simulink model "Cardiovs_Perez22210425"  (R2023a)
settings: Solver=ode15s  StartTime=0.0  StopTime=10  MaxStep=1e-3  RelTol=1e-3
settings Model: Creator=najap  LastModifiedBy=najap
settings DataIOCC: SaveOutput=off  ReturnWorkspaceOutputs=off  TimeSaveName=t
settings DebuggingCC: AlgebraicLoopMsg=none  ArtificialAlgebraicLoopMsg=none  MaxConsecutiveZCsMsg=none  SolverPrmCheckMsg=warning  ModelReferenceExtraNoncontSigs=none  OperatingPointInterfaceChecksumMismatchMsg=none

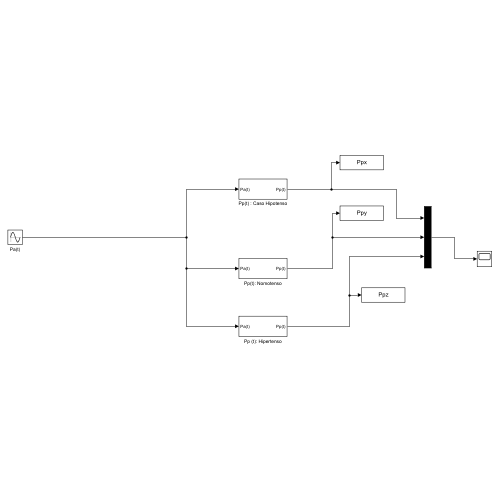
[thumbnail: Simulink's stored preview of the top-level diagram]
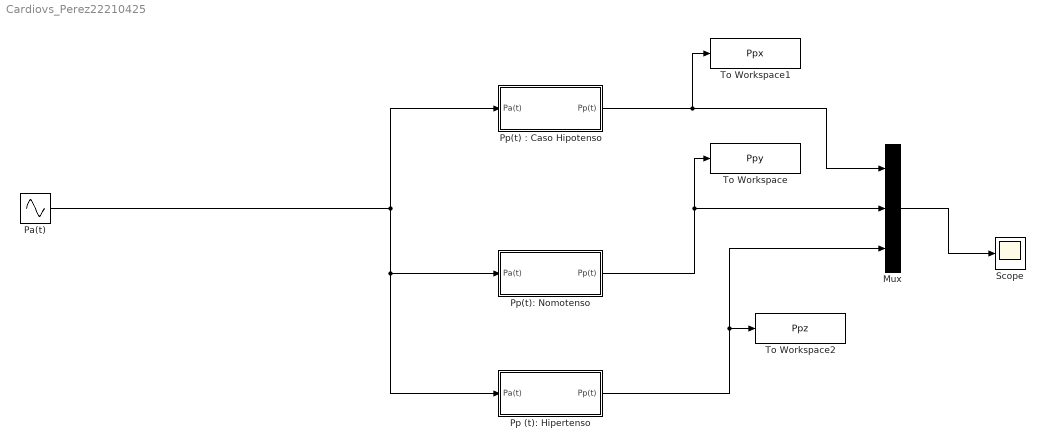
== system Cardiovs_Perez22210425 ==
  Mux : Mux  Inputs=3
  Pa(t) : Sin  Bias=0.8  Frequency=2*pi*95/60  SampleTime=0
  Pp (t): Hipertenso : Subsystem
  "Pp(t) : Caso Hipotenso" : Subsystem
  Pp(t): Nomotenso : Subsystem
  Scope : Scope
  To Workspace : ToWorkspace  VariableName=Ppy  SaveFormat=Timeseries  SampleTime=-1
  To Workspace1 : ToWorkspace  VariableName=Ppx  SaveFormat=Timeseries  SampleTime=-1
  To Workspace2 : ToWorkspace  VariableName=Ppz  SaveFormat=Timeseries  SampleTime=-1
  wires:
  Mux/1 -> Scope/1
  Pp (t): Hipertenso/1(Pp(t)) -> Mux/3, To Workspace2/1
  Pa(t)/1 -> Pp(t): Nomotenso/1(Pa(t)), Pp (t): Hipertenso/1(Pa(t)), "Pp(t) : Caso Hipotenso"/1(Pa(t))
  Pp(t): Nomotenso/1(Pp(t)) -> To Workspace/1, Mux/2
  "Pp(t) : Caso Hipotenso"/1(Pp(t)) -> To Workspace1/1, Mux/1

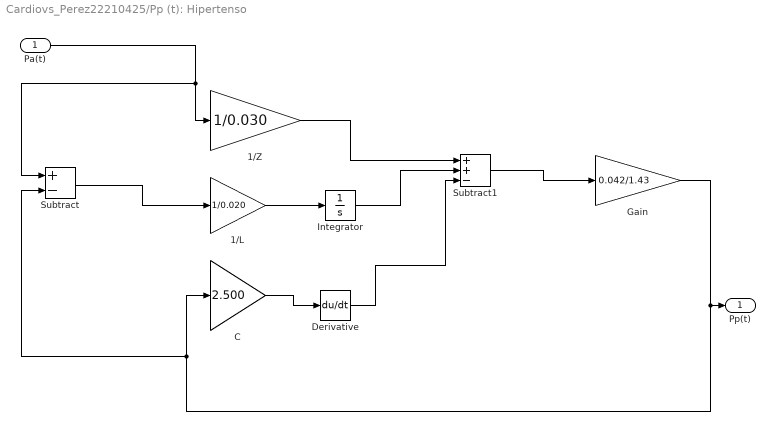
== system Cardiovs_Perez22210425/Pp (t): Hipertenso ==
  Pa(t) : Inport
  1/L : Gain  Gain=1/0.020
  1/Z : Gain  Gain=1/0.030
  C : Gain  Gain=2.500
  Derivative : Derivative
  Gain : Gain  Gain=0.042/1.43
  Integrator : Integrator
  Subtract : Sum  Inputs=+-
  Subtract1 : Sum  Inputs=++-
  Pp(t) : Outport
  wires:
  Gain/1 -> Pp(t)/1, Subtract/2, C/1
  1/Z/1 -> Subtract1/1
  Subtract1/1 -> Gain/1
  Integrator/1 -> Subtract1/2
  Subtract/1 -> 1/L/1
  1/L/1 -> Integrator/1
  Derivative/1 -> Subtract1/3
  C/1 -> Derivative/1
  Pa(t)/1 -> Subtract/1, 1/Z/1

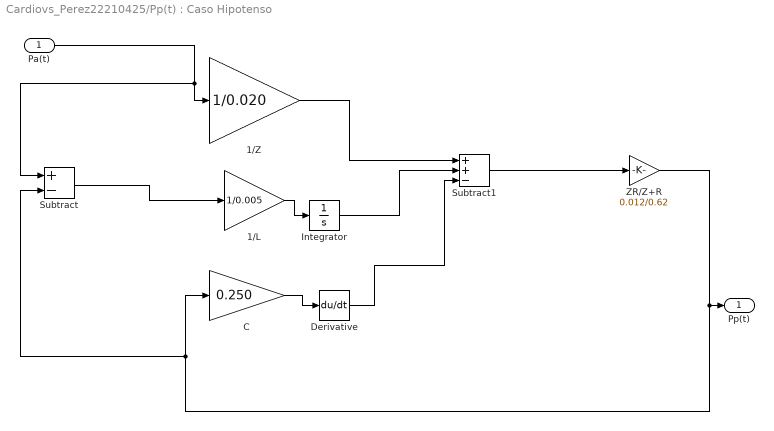
== system Cardiovs_Perez22210425/Pp(t) : Caso Hipotenso ==
  Pa(t) : Inport
  1/L : Gain  Gain=1/0.005
  1/Z : Gain  Gain=1/0.020
  C : Gain  Gain=0.250
  Derivative : Derivative
  Integrator : Integrator
  Subtract : Sum  Inputs=+-
  Subtract1 : Sum  Inputs=++-
  ZR/Z+R : Gain  Gain=0.012/0.62
  Pp(t) : Outport
  wires:
  C/1 -> Derivative/1
  1/L/1 -> Integrator/1
  Integrator/1 -> Subtract1/2
  1/Z/1 -> Subtract1/1
  Derivative/1 -> Subtract1/3
  Subtract/1 -> 1/L/1
  Pa(t)/1 -> Subtract/1, 1/Z/1
  Subtract1/1 -> ZR/Z+R/1
  ZR/Z+R/1 -> Subtract/2, C/1, Pp(t)/1

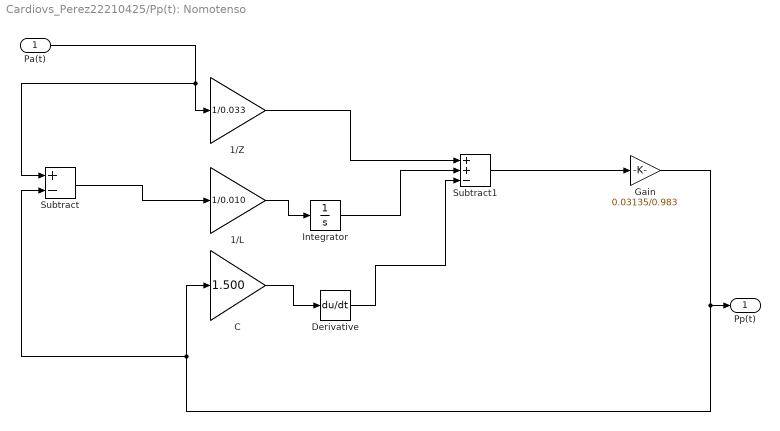
== system Cardiovs_Perez22210425/Pp(t): Nomotenso ==
  Pa(t) : Inport
  1/L : Gain  Gain=1/0.010
  1/Z : Gain  Gain=1/0.033
  C : Gain  Gain=1.500
  Derivative : Derivative
  Gain : Gain  Gain=0.03135/0.983
  Integrator : Integrator
  Subtract : Sum  Inputs=+-
  Subtract1 : Sum  Inputs=++-
  Pp(t) : Outport
  wires:
  Gain/1 -> Pp(t)/1, Subtract/2, C/1
  1/Z/1 -> Subtract1/1
  Subtract1/1 -> Gain/1
  Integrator/1 -> Subtract1/2
  Subtract/1 -> 1/L/1
  1/L/1 -> Integrator/1
  Derivative/1 -> Subtract1/3
  C/1 -> Derivative/1
  Pa(t)/1 -> Subtract/1, 1/Z/1
